simulink model "sampleModel1410"  (R2023a)
settings: Solver=VariableStepAuto  StartTime=0.0  StopTime=10.0  RelTol=1e-3
libraries: hdlsllib x4, simulink x1
settings Model: Creator=user1  LastModifiedBy=user1

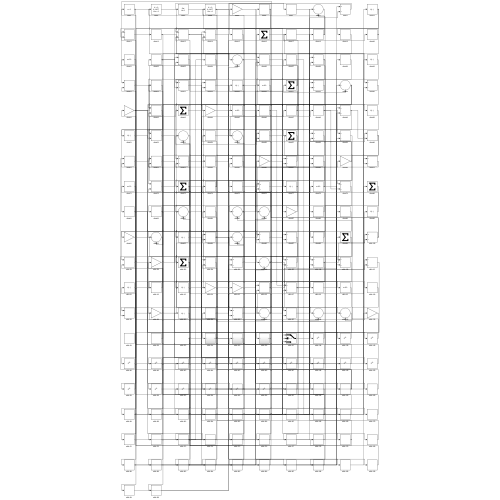
[thumbnail: Simulink's stored preview of the top-level diagram]
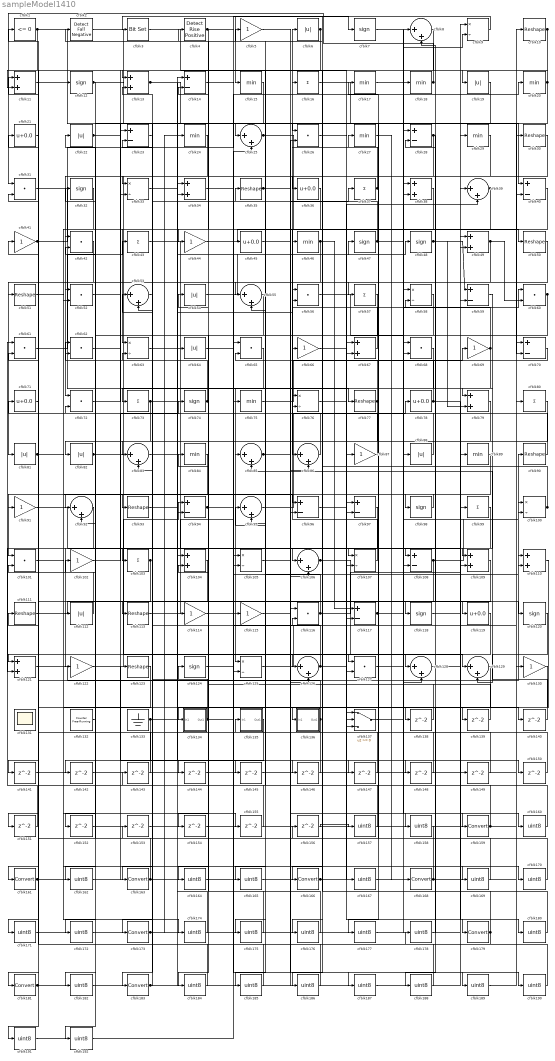
== system sampleModel1410 ==
  cfblk1 : hdlsllib/Logic and Bit Operations/Compare To Zero  relop=<=  OutDataTypeStr=boolean
  cfblk{10,30,35,50..51,77,90,93,111,113,123} (11 alike) : Reshape
  cfblk{9,33,58,63,76,100,105,107,125} (9 alike) : Product  Inputs=*/  RndMeth=Zero  SaturateOnIntegerOverflow=on
  cfblk{26,31,42,52,56,60..62,65,68,72,101,116,127} (14 alike) : DotProduct  OutDataTypeStr=Inherit: Inherit via internal rule
  cfblk{5,41,44,66,69,87,91,102,114..115,122,130} (12 alike) : Gain
  cfblk{16,37,43,57,73,80,99,103} (8 alike) : Sum  Inputs=+
  cfblk{11,13,34,38,49,67,79,104,109..110,121} (11 alike) : Sum
  cfblk{8,25,39,53,55,83,85..86,92,95,106,126,128..129} (14 alike) : Sum  Inputs=|++
  cfblk{14,23,28,40,59,70,94,96..97,108,117} (11 alike) : Sum  Inputs=+-
  cfblk{6,19,22,54,64,81..82,88,112} (9 alike) : Abs  SaturateOnIntegerOverflow=off
  cfblk{7,12,32,47..48,74,98,118,120,124} (10 alike) : Signum
  cfblk{21,36,45,71,78,119} (6 alike) : Bias  Bias=0.0  SaturateOnIntegerOverflow=off
  cfblk131 : Scope
      settings: Floating=on
  cfblk132 : hdlsllib/Sources/Counter Free-Running  NumBits=16  tsamp=-1
  cfblk133 : Ground
  cfblk134 : Subsystem
      settings: LibrarySourceBlock=|
      | hdlsllib/Ports &
      | Subsystems/Subsystem
  cfblk135 : Subsystem
      settings: LibrarySourceBlock=|
      | hdlsllib/Ports &
      | Subsystems/Subsystem
  cfblk136 : Subsystem
      settings: LibrarySourceBlock=|
      | hdlsllib/Ports &
      | Subsystems/Subsystem
  cfblk137 : Switch  SaturateOnIntegerOverflow=off  InputSameDT=off
  cfblk{138..156} (19 alike) : Delay  SampleTime=1
  cfblk{15,17..18,20,24,27,29,46,75,84,89} (11 alike) : MinMax
  cfblk{157..158,160,162,164..165,167,169..172,174..178,180,182,184..192} (27 alike) : DataTypeConversion  OutDataTypeStr=uint8  SaturateOnIntegerOverflow=off  RndMeth=Floor
  cfblk{159,161,163,166,168,173,179,181,183} (9 alike) : DataTypeConversion  SaturateOnIntegerOverflow=off  RndMeth=Floor
  cfblk2 : hdlsllib/Logic and Bit Operations/Detect Fall Negative  vinit=0  OutDataTypeStr=boolean
  cfblk3 : simulink/Logic and Bit Operations/Bit Set  iBit=0
      settings: LibrarySourceBlock=|
      | hdlsllib/Logic and Bit
      | Operations/Bit Set
  cfblk4 : hdlsllib/Logic and Bit Operations/Detect Rise Positive  vinit=0  OutDataTypeStr=boolean
  wires:
  cfblk43/1 -> cfblk108/1
  cfblk24/1 -> cfblk127/1
  cfblk122/1 -> cfblk94/1
  cfblk20/1 -> cfblk19/1, cfblk52/1
  cfblk107/1 -> cfblk6/1
  cfblk77/1 -> cfblk15/1, cfblk175/1
  cfblk49/1 -> cfblk81/1, cfblk60/2
  cfblk111/1 -> cfblk119/1
  cfblk80/1 -> cfblk118/1
  cfblk82/1 -> cfblk128/1, cfblk112/1
  cfblk95/1 -> cfblk78/1
  cfblk44/1 -> cfblk50/1
  cfblk18/1 -> cfblk31/1, cfblk13/1
  cfblk37/1 -> cfblk16/1, cfblk36/1
  cfblk22/1 -> cfblk26/1, cfblk139/1
  cfblk6/1 -> cfblk51/1, cfblk95/2
  cfblk121/1 -> cfblk90/1
  cfblk36/1 -> cfblk86/1
  cfblk2/1 -> cfblk25/1
  cfblk108/1 -> cfblk100/1, cfblk154/1
  cfblk104/1 -> cfblk173/1
  cfblk13/1 -> cfblk87/1, cfblk146/1
  cfblk68/1 -> cfblk163/1
  cfblk89/1 -> cfblk181/1
  cfblk35/1 -> cfblk55/1, cfblk158/1
  cfblk110/1 -> cfblk136/1(In1)
  cfblk64/1 -> cfblk25/2
  cfblk83/1 -> cfblk14/1
  cfblk39/1 -> cfblk63/1, cfblk92/1, cfblk52/2
  cfblk74/1 -> cfblk73/1, cfblk32/1
  cfblk1/1 -> cfblk40/1, cfblk11/2
  cfblk73/1 -> cfblk109/2, cfblk162/1
  cfblk56/1 -> cfblk128/2
  cfblk97/1 -> cfblk122/1
  cfblk86/1 -> cfblk54/1
  cfblk125/1 -> cfblk80/1
  cfblk137/1 -> cfblk18/1
  cfblk136/1(Out1) -> cfblk135/1(In1), cfblk11/1
  cfblk134/1(Out1) -> cfblk110/1, cfblk23/2, cfblk150/1
  cfblk126/1 -> cfblk67/2, cfblk83/2, cfblk56/1
  cfblk55/1 -> cfblk134/1(In1)
  cfblk65/1 -> cfblk125/1
  cfblk112/1 -> cfblk71/1
  cfblk60/1 -> cfblk109/1, cfblk165/1
  cfblk78/1 -> cfblk55/2, cfblk180/1
  cfblk30/1 -> cfblk166/1
  cfblk23/1 -> cfblk103/1
  cfblk98/1 -> cfblk93/1
  cfblk67/1 -> cfblk46/1
  cfblk96/1 -> cfblk69/1
  cfblk84/1 -> cfblk101/1
  cfblk116/1 -> cfblk35/1, cfblk59/2
  cfblk132/1 -> cfblk102/1
  cfblk106/1 -> cfblk129/1, cfblk39/2
  cfblk45/1 -> cfblk120/1
  cfblk113/1 -> cfblk45/1
  cfblk71/1 -> cfblk91/1
  cfblk120/1 -> cfblk129/2
  cfblk40/1 -> cfblk126/1
  cfblk66/1 -> cfblk179/1
  cfblk50/1 -> cfblk94/2
  cfblk117/1 -> cfblk100/2, cfblk9/2
  cfblk72/1 -> cfblk23/1
  cfblk61/1 -> cfblk43/1
  cfblk33/1 -> cfblk114/1
  cfblk41/1 -> cfblk20/1, cfblk155/1, cfblk174/1
  cfblk29/1 -> cfblk72/1
  cfblk9/1 -> cfblk3/1
  cfblk100/1 -> cfblk2/1, cfblk76/1
  cfblk17/1 -> cfblk58/1
  cfblk31/1 -> cfblk125/2
  cfblk25/1 -> cfblk85/1, cfblk107/2
  cfblk133/1 -> cfblk56/2, cfblk182/1, cfblk192/1
  cfblk115/1 -> cfblk110/2
  cfblk11/1 -> cfblk12/1
  cfblk70/1 -> cfblk65/2
  cfblk63/1 -> cfblk47/1
  cfblk91/1 -> cfblk106/1
  cfblk90/1 -> cfblk21/1
  cfblk102/1 -> cfblk74/1
  cfblk57/1 -> cfblk82/1
  cfblk53/1 -> cfblk183/1
  cfblk75/1 -> cfblk28/1
  cfblk114/1 -> cfblk115/1
  cfblk118/1 -> cfblk9/1
  cfblk124/1 -> cfblk116/2
  cfblk16/1 -> cfblk70/2
  cfblk127/1 -> cfblk60/1
  cfblk4/1 -> cfblk44/1, cfblk7/1, cfblk77/1
  cfblk28/1 -> cfblk57/1, cfblk98/1
  cfblk3/1 -> cfblk97/2
  cfblk123/1 -> cfblk161/1
  cfblk103/1 -> cfblk113/1, cfblk191/1
  cfblk32/1 -> cfblk42/1
  cfblk88/1 -> cfblk62/1
  cfblk47/1 -> cfblk88/1, cfblk13/2
  cfblk12/1 -> cfblk75/1, cfblk92/2
  cfblk81/1 -> cfblk96/1, cfblk137/2
  cfblk54/1 -> cfblk48/1
  cfblk59/1 -> cfblk79/1
  cfblk5/1 -> cfblk159/1
  cfblk94/1 -> cfblk107/1, cfblk189/1
  cfblk58/1 -> cfblk83/1
  cfblk48/1 -> cfblk59/1, cfblk79/2
  cfblk46/1 -> cfblk96/2, cfblk117/1
  cfblk87/1 -> cfblk62/2
  cfblk15/1 -> cfblk33/1
  cfblk27/1 -> cfblk168/1
  cfblk69/1 -> cfblk17/1, cfblk28/2, cfblk184/1
  cfblk128/1 -> cfblk29/1
  cfblk85/1 -> cfblk37/1, cfblk185/1
  cfblk10/1 -> cfblk121/1, cfblk33/2
  cfblk92/1 -> cfblk121/2
  cfblk51/1 -> cfblk138/1
  cfblk138/1 -> cfblk14/2
  cfblk139/1 -> cfblk67/1
  cfblk26/1 -> cfblk140/1
  cfblk140/1 -> cfblk85/2
  cfblk21/1 -> cfblk141/1
  cfblk141/1 -> cfblk97/1
  cfblk135/1(Out1) -> cfblk142/1
  cfblk142/1 -> cfblk70/1
  cfblk143/1 -> cfblk72/2
  cfblk129/1 -> cfblk144/1
  cfblk144/1 -> cfblk65/1
  cfblk62/1 -> cfblk145/1
  cfblk145/1 -> cfblk39/1
  cfblk146/1 -> cfblk63/2
  cfblk52/1 -> cfblk147/1
  cfblk147/1 -> cfblk95/1
  cfblk93/1 -> cfblk148/1
  cfblk148/1 -> cfblk1/1
  cfblk149/1 -> cfblk101/2
  cfblk150/1 -> cfblk58/2
  cfblk119/1 -> cfblk151/1
  cfblk151/1 -> cfblk61/1
  cfblk79/1 -> cfblk152/1
  cfblk152/1 -> cfblk108/2
  cfblk153/1 -> cfblk126/2
  cfblk154/1 -> cfblk40/2
  cfblk155/1 -> cfblk4/1
  cfblk156/1 -> cfblk157/1
  cfblk157/1 -> cfblk116/1
  cfblk158/1 -> cfblk156/1
  cfblk159/1 -> cfblk137/1, cfblk124/1, cfblk41/1
  cfblk7/1 -> cfblk160/1
  cfblk160/1 -> cfblk5/1
  cfblk161/1 -> cfblk137/3, cfblk127/2
  cfblk162/1 -> cfblk123/1
  cfblk163/1 -> cfblk117/2, cfblk38/2, cfblk31/2
  cfblk109/1 -> cfblk164/1
  cfblk164/1 -> cfblk68/1
  cfblk165/1 -> cfblk68/2
  cfblk166/1 -> cfblk149/1, cfblk10/1
  cfblk76/1 -> cfblk167/1
  cfblk167/1 -> cfblk30/1
  cfblk168/1 -> cfblk76/2, cfblk42/2
  cfblk101/1 -> cfblk169/1
  cfblk169/1 -> cfblk27/1
  cfblk34/1 -> cfblk170/1
  cfblk170/1 -> cfblk22/1
  cfblk42/1 -> cfblk171/1
  cfblk171/1 -> cfblk34/1
  cfblk38/1 -> cfblk172/1
  cfblk172/1 -> cfblk34/2
  cfblk173/1 -> cfblk49/1, cfblk26/2, cfblk24/1
  cfblk174/1 -> cfblk104/1
  cfblk175/1 -> cfblk104/2
  cfblk8/1 -> cfblk176/1
  cfblk176/1 -> cfblk84/1
  cfblk19/1 -> cfblk177/1
  cfblk177/1 -> cfblk8/1
  cfblk178/1 -> cfblk8/2
  cfblk179/1 -> cfblk178/1, cfblk38/1
  cfblk180/1 -> cfblk66/1
  cfblk181/1 -> cfblk49/2, cfblk64/1
  cfblk182/1 -> cfblk89/1
  cfblk183/1 -> cfblk153/1, cfblk106/2, cfblk86/2
  cfblk184/1 -> cfblk53/1
  cfblk185/1 -> cfblk53/2
  cfblk99/1 -> cfblk186/1
  cfblk186/1 -> cfblk61/2
  cfblk14/1 -> cfblk187/1
  cfblk187/1 -> cfblk99/1
  cfblk130/1 -> cfblk188/1
  cfblk188/1 -> cfblk111/1
  cfblk189/1 -> cfblk130/1
  cfblk105/1 -> cfblk190/1
  cfblk190/1 -> cfblk143/1
  cfblk191/1 -> cfblk105/1
  cfblk192/1 -> cfblk105/2

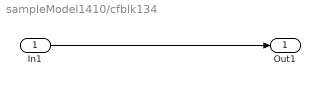
== system sampleModel1410/cfblk134 ==
  In1 : Inport
  Out1 : Outport
  wires:
  In1/1 -> Out1/1

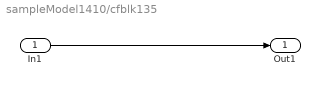
== system sampleModel1410/cfblk135 ==
  In1 : Inport
  Out1 : Outport
  wires:
  In1/1 -> Out1/1

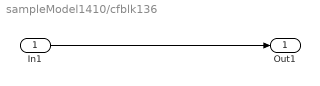
== system sampleModel1410/cfblk136 ==
  In1 : Inport
  Out1 : Outport
  wires:
  In1/1 -> Out1/1
